simulink library "halin"  (R2021b)
settings: Solver=VariableStepAuto  StartTime=0.0  StopTime=10.0  RelTol=1e-3
undefined symbols (not defined in the file): KHAL_CAN1ABM1E2E_flg, KHAL_CAN1ESC1E2E_flg, KHAL_CAN1ESC5E2E_flg, KHAL_CAN1ESC7E2E_flg, KHAL_CAN1FCM2E2E_flg, KHAL_CAN1FCM3E2E_flg, KHAL_CAN1FCM4E2E_flg, KHAL_CAN3BMS1E2E_flg, KHAL_CAN3BMS6E2E_flg, KHAL_CAN3CCU1E2E_flg, KHAL_CAN3CCU2E2E_flg, KHAL_CAN3MCUF1E2E_flg, KHAL_CAN3MCUR1E2E_flg, KHAL_CAN3Shifter1E2E_flg, TRUE
libraries: simulink x420, FVT_lib x149, hcu_lib x49
(part 11 of 14)

== system halin/HAL_IN/CAN4/GW_ZoneDR1 ==
  DT_CAN4_SG_GW_ZoneDR1 : Inport
  CSWDimSw : Subsystem
  CSWFWasSwSta : Subsystem
  CSWFWipSwSta : Subsystem
  CSWPassSWSta : Subsystem
  CSWRWasSWSta : Subsystem
  CSWRWipIntSwSta : Subsystem
  CSWTurnSwSta : Subsystem
  DrLockSta : Subsystem
  MIRRORFOLDSW : Subsystem
  RLSLampSta : Subsystem
  RLSRainSnrWiperCmd : Subsystem
  RLTurnLampC : Subsystem
  RRTurnLampC : Subsystem
  RWiperAS : Subsystem
  RWiperProtection : Subsystem
  bus_selector : BusSelector  OutputSignals=CAN4_CSW_DimSw
  bus_selector1 : BusSelector  OutputSignals=CAN4_CSW_FWasSw_Sta
  bus_selector10 : BusSelector  OutputSignals=CAN4_RLS_RainSnrWiperCmd
  bus_selector11 : BusSelector  OutputSignals=CAN4_RLTurnLampC
  bus_selector12 : BusSelector  OutputSignals=CAN4_RRTurnLampC
  bus_selector13 : BusSelector  OutputSignals=CAN4_RWiperAS
  bus_selector14 : BusSelector  OutputSignals=CAN4_RWiperProtection
  bus_selector2 : BusSelector  OutputSignals=CAN4_CSW_FWipSw_Sta
  bus_selector3 : BusSelector  OutputSignals=CAN4_CSW_PassSW_Sta
  bus_selector4 : BusSelector  OutputSignals=CAN4_CSW_RWasSW_Sta
  bus_selector5 : BusSelector  OutputSignals=CAN4_CSW_RWipIntSw_Sta
  bus_selector6 : BusSelector  OutputSignals=CAN4_CSW_TurnSw_Sta
  bus_selector7 : BusSelector  OutputSignals=CAN4_DrLockSta
  bus_selector8 : BusSelector  OutputSignals=CAN4_MIRROR_FOLD_SW
  bus_selector9 : BusSelector  OutputSignals=CAN4_RLS_Lamp_Sta
  VHAL_CSWDimSw_flg : Outport
  VHAL_CSWFWasSwSta_enum : Outport  Port=2
  VHAL_CSWFWipSwSta_enum : Outport  Port=3
  VHAL_CSWPassSWSta_flg : Outport  Port=4
  VHAL_CSWRWasSWSta_enum : Outport  Port=5
  VHAL_CSWRWipIntSwSta_enum : Outport  Port=6
  VHAL_CSWTurnSwSta_enum : Outport  Port=7
  VHAL_DrLockSta_flg : Outport  Port=8
  VHAL_MIRRORFOLDSW_flg : Outport  Port=9
  VHAL_RLSLampSta_flg : Outport  Port=10
  VHAL_RLSRainSnrWiperCmd_enum : Outport  Port=11
  VHAL_RLTurnLampC_mA : Outport  Port=12
  VHAL_RRTurnLampC_mA : Outport  Port=13
  VHAL_RWiperAS_flg : Outport  Port=14
  VHAL_RWiperProtection_flg : Outport  Port=15
  wires:
  DT_CAN4_SG_GW_ZoneDR1/1 -> [DT_CAN4_SG_GW_ZoneDR1]
  [DT_CAN4_SG_GW_ZoneDR1] -> bus_selector/1
  bus_selector/1 -> CSWDimSw/1(CSW_DimSw)  "<CAN4_CSW_DimSw>"
  CSWDimSw/1(VHAL_CSWDimSw_flg) -> VHAL_CSWDimSw_flg/1
  [DT_CAN4_SG_GW_ZoneDR1] -> bus_selector1/1
  bus_selector1/1 -> CSWFWasSwSta/1(CSW_FWasSw_Sta)  "<CAN4_CSW_FWasSw_Sta>"
  CSWFWasSwSta/1(VHAL_CSWFWasSwSta_enum) -> VHAL_CSWFWasSwSta_enum/1
  [DT_CAN4_SG_GW_ZoneDR1] -> bus_selector2/1
  bus_selector2/1 -> CSWFWipSwSta/1(CSW_FWipSw_Sta)  "<CAN4_CSW_FWipSw_Sta>"
  CSWFWipSwSta/1(VHAL_CSWFWipSwSta_enum) -> VHAL_CSWFWipSwSta_enum/1
  [DT_CAN4_SG_GW_ZoneDR1] -> bus_selector3/1
  bus_selector3/1 -> CSWPassSWSta/1(CSW_PassSW_Sta)  "<CAN4_CSW_PassSW_Sta>"
  CSWPassSWSta/1(VHAL_CSWPassSWSta_flg) -> VHAL_CSWPassSWSta_flg/1
  [DT_CAN4_SG_GW_ZoneDR1] -> bus_selector4/1
  bus_selector4/1 -> CSWRWasSWSta/1(CSW_RWasSW_Sta)  "<CAN4_CSW_RWasSW_Sta>"
  CSWRWasSWSta/1(VHAL_CSWRWasSWSta_enum) -> VHAL_CSWRWasSWSta_enum/1
  [DT_CAN4_SG_GW_ZoneDR1] -> bus_selector5/1
  bus_selector5/1 -> CSWRWipIntSwSta/1(CSW_RWipIntSw_Sta)  "<CAN4_CSW_RWipIntSw_Sta>"
  CSWRWipIntSwSta/1(VHAL_CSWRWipIntSwSta_enum) -> VHAL_CSWRWipIntSwSta_enum/1
  [DT_CAN4_SG_GW_ZoneDR1] -> bus_selector6/1
  bus_selector6/1 -> CSWTurnSwSta/1(CSW_TurnSw_Sta)  "<CAN4_CSW_TurnSw_Sta>"
  CSWTurnSwSta/1(VHAL_CSWTurnSwSta_enum) -> VHAL_CSWTurnSwSta_enum/1
  [DT_CAN4_SG_GW_ZoneDR1] -> bus_selector7/1
  bus_selector7/1 -> DrLockSta/1(DrLockSta)  "<CAN4_DrLockSta>"
  DrLockSta/1(VHAL_DrLockSta_flg) -> VHAL_DrLockSta_flg/1
  [DT_CAN4_SG_GW_ZoneDR1] -> bus_selector8/1
  bus_selector8/1 -> MIRRORFOLDSW/1(MIRROR_FOLD_SW)  "<CAN4_MIRROR_FOLD_SW>"
  MIRRORFOLDSW/1(VHAL_MIRRORFOLDSW_flg) -> VHAL_MIRRORFOLDSW_flg/1
  [DT_CAN4_SG_GW_ZoneDR1] -> bus_selector9/1
  bus_selector9/1 -> RLSLampSta/1(RLS_Lamp_Sta)  "<CAN4_RLS_Lamp_Sta>"
  RLSLampSta/1(VHAL_RLSLampSta_flg) -> VHAL_RLSLampSta_flg/1
  [DT_CAN4_SG_GW_ZoneDR1] -> bus_selector10/1
  bus_selector10/1 -> RLSRainSnrWiperCmd/1(RLS_RainSnrWiperCmd)  "<CAN4_RLS_RainSnrWiperCmd>"
  RLSRainSnrWiperCmd/1(VHAL_RLSRainSnrWiperCmd_enum) -> VHAL_RLSRainSnrWiperCmd_enum/1
  [DT_CAN4_SG_GW_ZoneDR1] -> bus_selector11/1
  bus_selector11/1 -> RLTurnLampC/1(RLTurnLampC)  "<CAN4_RLTurnLampC>"
  RLTurnLampC/1(VHAL_RLTurnLampC_mA) -> VHAL_RLTurnLampC_mA/1
  [DT_CAN4_SG_GW_ZoneDR1] -> bus_selector12/1
  bus_selector12/1 -> RRTurnLampC/1(RRTurnLampC)  "<CAN4_RRTurnLampC>"
  RRTurnLampC/1(VHAL_RRTurnLampC_mA) -> VHAL_RRTurnLampC_mA/1
  [DT_CAN4_SG_GW_ZoneDR1] -> bus_selector13/1
  bus_selector13/1 -> RWiperAS/1(RWiperAS)  "<CAN4_RWiperAS>"
  RWiperAS/1(VHAL_RWiperAS_flg) -> VHAL_RWiperAS_flg/1
  [DT_CAN4_SG_GW_ZoneDR1] -> bus_selector14/1
  bus_selector14/1 -> RWiperProtection/1(RWiperProtection)  "<CAN4_RWiperProtection>"
  RWiperProtection/1(VHAL_RWiperProtection_flg) -> VHAL_RWiperProtection_flg/1

== system halin/HAL_IN/CAN4/GW_ZoneDR2 ==
  DT_CAN4_SG_GW_ZoneDR2 : Inport
  SWCCANCELSta : Subsystem
  SWCResUpSta : Subsystem
  SWCSetdownSta : Subsystem
  SWCmodeSta : Subsystem
  bus_selector : BusSelector  OutputSignals=CAN4_SWC_CANCEL_Sta
  bus_selector1 : BusSelector  OutputSignals=CAN4_SWC_Res_Up_Sta
  bus_selector2 : BusSelector  OutputSignals=CAN4_SWC_Set_down_Sta
  bus_selector3 : BusSelector  OutputSignals=CAN4_SWC_mode_Sta
  VHAL_SWCCANCELSta_flg : Outport
  VHAL_SWCResUpSta_flg : Outport  Port=2
  VHAL_SWCSetdownSta_flg : Outport  Port=3
  VHAL_SWCmodeSta_flg : Outport  Port=4
  wires:
  DT_CAN4_SG_GW_ZoneDR2/1 -> [DT_CAN4_SG_GW_ZoneDR2]
  [DT_CAN4_SG_GW_ZoneDR2] -> bus_selector/1
  bus_selector/1 -> SWCCANCELSta/1(SWC_CANCEL_Sta)  "<CAN4_SWC_CANCEL_Sta>"
  SWCCANCELSta/1(VHAL_SWCCANCELSta_flg) -> VHAL_SWCCANCELSta_flg/1
  [DT_CAN4_SG_GW_ZoneDR2] -> bus_selector1/1
  bus_selector1/1 -> SWCResUpSta/1(SWC_Res_Up_Sta)  "<CAN4_SWC_Res_Up_Sta>"
  SWCResUpSta/1(VHAL_SWCResUpSta_flg) -> VHAL_SWCResUpSta_flg/1
  [DT_CAN4_SG_GW_ZoneDR2] -> bus_selector2/1
  bus_selector2/1 -> SWCSetdownSta/1(SWC_Set_down_Sta)  "<CAN4_SWC_Set_down_Sta>"
  SWCSetdownSta/1(VHAL_SWCSetdownSta_flg) -> VHAL_SWCSetdownSta_flg/1
  [DT_CAN4_SG_GW_ZoneDR2] -> bus_selector3/1
  bus_selector3/1 -> SWCmodeSta/1(SWC_mode_Sta)  "<CAN4_SWC_mode_Sta>"
  SWCmodeSta/1(VHAL_SWCmodeSta_flg) -> VHAL_SWCmodeSta_flg/1

== system halin/HAL_IN/CAN4/GW_ZoneDR3 ==
  DT_CAN4_SG_GW_ZoneDR3 : Inport
  LDrvValWdwOpened : Subsystem
  LPasValWdwOpened : Subsystem
  bus_selector : BusSelector  OutputSignals=CAN4_L_Drv_Val_Wdw_Opened
  bus_selector1 : BusSelector  OutputSignals=CAN4_L_Pas_Val_Wdw_Opened
  VHAL_LDrvValWdwOpened_pct : Outport
  VHAL_LPasValWdwOpened_pct : Outport  Port=2
  wires:
  DT_CAN4_SG_GW_ZoneDR3/1 -> [DT_CAN4_SG_GW_ZoneDR3]
  [DT_CAN4_SG_GW_ZoneDR3] -> bus_selector/1
  bus_selector/1 -> LDrvValWdwOpened/1(L_Drv_Val_Wdw_Opened)  "<CAN4_L_Drv_Val_Wdw_Opened>"
  LDrvValWdwOpened/1(VHAL_LDrvValWdwOpened_pct) -> VHAL_LDrvValWdwOpened_pct/1
  [DT_CAN4_SG_GW_ZoneDR3] -> bus_selector1/1
  bus_selector1/1 -> LPasValWdwOpened/1(L_Pas_Val_Wdw_Opened)  "<CAN4_L_Pas_Val_Wdw_Opened>"
  LPasValWdwOpened/1(VHAL_LPasValWdwOpened_pct) -> VHAL_LPasValWdwOpened_pct/1

== system halin/HAL_IN/CAN4/GW_ZoneDR4 ==
  DT_CAN4_SG_GW_ZoneDR4 : Inport
  LRLDValWdwOpened : Subsystem
  LRRDValWdwOpened : Subsystem
  PTGInnerSW2 : Subsystem
  bus_selector : BusSelector  OutputSignals=CAN4_L_RLD_Val_Wdw_Opened
  bus_selector1 : BusSelector  OutputSignals=CAN4_L_RRD_Val_Wdw_Opened
  bus_selector2 : BusSelector  OutputSignals=CAN4_PTG_Inner_SW_2
  VHAL_LRLDValWdwOpened_pct : Outport
  VHAL_LRRDValWdwOpened_pct : Outport  Port=2
  VHAL_PTGInnerSW2_enum : Outport  Port=3
  wires:
  DT_CAN4_SG_GW_ZoneDR4/1 -> [DT_CAN4_SG_GW_ZoneDR4]
  [DT_CAN4_SG_GW_ZoneDR4] -> bus_selector/1
  bus_selector/1 -> LRLDValWdwOpened/1(L_RLD_Val_Wdw_Opened)  "<CAN4_L_RLD_Val_Wdw_Opened>"
  LRLDValWdwOpened/1(VHAL_LRLDValWdwOpened_pct) -> VHAL_LRLDValWdwOpened_pct/1
  [DT_CAN4_SG_GW_ZoneDR4] -> bus_selector1/1
  bus_selector1/1 -> LRRDValWdwOpened/1(L_RRD_Val_Wdw_Opened)  "<CAN4_L_RRD_Val_Wdw_Opened>"
  LRRDValWdwOpened/1(VHAL_LRRDValWdwOpened_pct) -> VHAL_LRRDValWdwOpened_pct/1
  [DT_CAN4_SG_GW_ZoneDR4] -> bus_selector2/1
  bus_selector2/1 -> PTGInnerSW2/1(PTG_Inner_SW_2)  "<CAN4_PTG_Inner_SW_2>"
  PTGInnerSW2/1(VHAL_PTGInnerSW2_enum) -> VHAL_PTGInnerSW2_enum/1

== system halin/HAL_IN/CAN4/GW_ZoneDR6 ==
  DT_CAN4_SG_GW_ZoneDR6 : Inport
  FrntPTCRearLeActHeatPwr : Subsystem
  FrntPTCRearRiActHeatPwr : Subsystem
  FrntPTCRiActHeatPwr : Subsystem
  bus_selector : BusSelector  OutputSignals=CAN4_FrntPTCRearLeActHeatPwr
  bus_selector1 : BusSelector  OutputSignals=CAN4_FrntPTCRearRiActHeatPwr
  bus_selector2 : BusSelector  OutputSignals=CAN4_FrntPTCRiActHeatPwr
  VHAL_FrntPTCRearLeActHeatPwr_W : Outport
  VHAL_FrntPTCRearRiActHeatPwr_W : Outport  Port=2
  VHAL_FrntPTCRiActHeatPwr_W : Outport  Port=3
  wires:
  DT_CAN4_SG_GW_ZoneDR6/1 -> [DT_CAN4_SG_GW_ZoneDR6]
  [DT_CAN4_SG_GW_ZoneDR6] -> bus_selector/1
  bus_selector/1 -> FrntPTCRearLeActHeatPwr/1(FrntPTCRearLeActHeatPwr)  "<CAN4_FrntPTCRearLeActHeatPwr>"
  FrntPTCRearLeActHeatPwr/1(VHAL_FrntPTCRearLeActHeatPwr_W) -> VHAL_FrntPTCRearLeActHeatPwr_W/1
  [DT_CAN4_SG_GW_ZoneDR6] -> bus_selector1/1
  bus_selector1/1 -> FrntPTCRearRiActHeatPwr/1(FrntPTCRearRiActHeatPwr)  "<CAN4_FrntPTCRearRiActHeatPwr>"
  FrntPTCRearRiActHeatPwr/1(VHAL_FrntPTCRearRiActHeatPwr_W) -> VHAL_FrntPTCRearRiActHeatPwr_W/1
  [DT_CAN4_SG_GW_ZoneDR6] -> bus_selector2/1
  bus_selector2/1 -> FrntPTCRiActHeatPwr/1(FrntPTCRiActHeatPwr)  "<CAN4_FrntPTCRiActHeatPwr>"
  FrntPTCRiActHeatPwr/1(VHAL_FrntPTCRiActHeatPwr_W) -> VHAL_FrntPTCRiActHeatPwr_W/1

== system halin/HAL_IN/CAN4/GW_ZoneFR1 ==
  DT_CAN4_SG_GW_ZoneFR1 : Inport
  FLTurnLampC : Subsystem
  FRTurnLampC : Subsystem
  FWiperAS : Subsystem
  FWiperProtection : Subsystem
  bus_selector : BusSelector  OutputSignals=CAN4_FLTurnLampC
  bus_selector1 : BusSelector  OutputSignals=CAN4_FRTurnLampC
  bus_selector2 : BusSelector  OutputSignals=CAN4_FWiperAS
  bus_selector3 : BusSelector  OutputSignals=CAN4_FWiperProtection
  VHAL_FLTurnLampC_mA : Outport
  VHAL_FRTurnLampC_mA : Outport  Port=2
  VHAL_FWiperAS_flg : Outport  Port=3
  VHAL_FWiperProtection_flg : Outport  Port=4
  wires:
  DT_CAN4_SG_GW_ZoneFR1/1 -> [DT_CAN4_SG_GW_ZoneFR1]
  [DT_CAN4_SG_GW_ZoneFR1] -> bus_selector/1
  bus_selector/1 -> FLTurnLampC/1(FLTurnLampC)  "<CAN4_FLTurnLampC>"
  FLTurnLampC/1(VHAL_FLTurnLampC_mA) -> VHAL_FLTurnLampC_mA/1
  [DT_CAN4_SG_GW_ZoneFR1] -> bus_selector1/1
  bus_selector1/1 -> FRTurnLampC/1(FRTurnLampC)  "<CAN4_FRTurnLampC>"
  FRTurnLampC/1(VHAL_FRTurnLampC_mA) -> VHAL_FRTurnLampC_mA/1
  [DT_CAN4_SG_GW_ZoneFR1] -> bus_selector2/1
  bus_selector2/1 -> FWiperAS/1(FWiperAS)  "<CAN4_FWiperAS>"
  FWiperAS/1(VHAL_FWiperAS_flg) -> VHAL_FWiperAS_flg/1
  [DT_CAN4_SG_GW_ZoneFR1] -> bus_selector3/1
  bus_selector3/1 -> FWiperProtection/1(FWiperProtection)  "<CAN4_FWiperProtection>"
  FWiperProtection/1(VHAL_FWiperProtection_flg) -> VHAL_FWiperProtection_flg/1

== system halin/HAL_IN/CAN4/GW_ZoneFR2 ==
  DT_CAN4_SG_GW_ZoneFR2 : Inport
  COMPStatorSpd : Subsystem
  CompProEN : Subsystem
  bus_selector : BusSelector  OutputSignals=CAN4_COMP_StatorSpd
  bus_selector1 : BusSelector  OutputSignals=CAN4_CompProEN
  VHAL_COMPStatorSpd_rpm : Outport
  VHAL_CompProEN_flg : Outport  Port=2
  wires:
  DT_CAN4_SG_GW_ZoneFR2/1 -> [DT_CAN4_SG_GW_ZoneFR2]
  [DT_CAN4_SG_GW_ZoneFR2] -> bus_selector/1
  bus_selector/1 -> COMPStatorSpd/1(COMP_StatorSpd)  "<CAN4_COMP_StatorSpd>"
  COMPStatorSpd/1(VHAL_COMPStatorSpd_rpm) -> VHAL_COMPStatorSpd_rpm/1
  [DT_CAN4_SG_GW_ZoneFR2] -> bus_selector1/1
  bus_selector1/1 -> CompProEN/1(CompProEN)  "<CAN4_CompProEN>"
  CompProEN/1(VHAL_CompProEN_flg) -> VHAL_CompProEN_flg/1

== system halin/HAL_IN/CAN4/VHAL_CANMsgInvalidDKC1_flg ==
  Cast To Boolean13 : DataTypeConversion  OutDataTypeStr=boolean
  Constant : Constant  Value=TRUE
  Latch13 : hcu_lib/Basic_Blocks/Latch
  Switch13 : Switch  Criteria=u2 ~= 0
  Unit Delay : UnitDelay  SampleTime=-1  HasFrameUpgradeWarning=on
  UnitConverter : DataTypeConversion  OutDataTypeStr=boolean
  Out : Outport
  wires:
  Constant/1 -> Switch13/3
  Unit Delay/1 -> Cast To Boolean13/1
  Cast To Boolean13/1 -> Switch13/1, Latch13/1
  Switch13/1 -> UnitConverter/1
  Latch13/1 -> Switch13/2
  UnitConverter/1 -> Unit Delay/1, Out/1  "VHAL_CANMsgInvalidDKC1_flg"

== system halin/HAL_IN/CAN4/VHAL_CANMsgInvalidDKC2_flg ==
  Cast To Boolean13 : DataTypeConversion  OutDataTypeStr=boolean
  Constant : Constant  Value=TRUE
  Latch13 : hcu_lib/Basic_Blocks/Latch
  Switch13 : Switch  Criteria=u2 ~= 0
  Unit Delay : UnitDelay  SampleTime=-1  HasFrameUpgradeWarning=on
  UnitConverter : DataTypeConversion  OutDataTypeStr=boolean
  Out : Outport
  wires:
  Constant/1 -> Switch13/3
  Unit Delay/1 -> Cast To Boolean13/1
  Cast To Boolean13/1 -> Switch13/1, Latch13/1
  Switch13/1 -> UnitConverter/1
  Latch13/1 -> Switch13/2
  UnitConverter/1 -> Unit Delay/1, Out/1  "VHAL_CANMsgInvalidDKC2_flg"

== system halin/HAL_IN/CAN4/VHAL_CANMsgInvalidGWZDRPTG1_flg ==
  Cast To Boolean13 : DataTypeConversion  OutDataTypeStr=boolean
  Constant : Constant  Value=TRUE
  Latch13 : hcu_lib/Basic_Blocks/Latch
  Switch13 : Switch  Criteria=u2 ~= 0
  Unit Delay : UnitDelay  SampleTime=-1  HasFrameUpgradeWarning=on
  UnitConverter : DataTypeConversion  OutDataTypeStr=boolean
  Out : Outport
  wires:
  Constant/1 -> Switch13/3
  Unit Delay/1 -> Cast To Boolean13/1
  Cast To Boolean13/1 -> Switch13/1, Latch13/1
  Switch13/1 -> UnitConverter/1
  Latch13/1 -> Switch13/2
  UnitConverter/1 -> Unit Delay/1, Out/1  "VHAL_CANMsgInvalidGWZDRPTG1_flg"

== system halin/HAL_IN/CAN4/VHAL_CANMsgInvalidGWZoneDR1_flg ==
  Cast To Boolean13 : DataTypeConversion  OutDataTypeStr=boolean
  Constant : Constant  Value=TRUE
  Latch13 : hcu_lib/Basic_Blocks/Latch
  Switch13 : Switch  Criteria=u2 ~= 0
  Unit Delay : UnitDelay  SampleTime=-1  HasFrameUpgradeWarning=on
  UnitConverter : DataTypeConversion  OutDataTypeStr=boolean
  Out : Outport
  wires:
  Constant/1 -> Switch13/3
  Unit Delay/1 -> Cast To Boolean13/1
  Cast To Boolean13/1 -> Switch13/1, Latch13/1
  Switch13/1 -> UnitConverter/1
  Latch13/1 -> Switch13/2
  UnitConverter/1 -> Unit Delay/1, Out/1  "VHAL_CANMsgInvalidGWZoneDR1_flg"

== system halin/HAL_IN/CAN4/VHAL_CANMsgInvalidGWZoneDR2_flg ==
  Cast To Boolean13 : DataTypeConversion  OutDataTypeStr=boolean
  Constant : Constant  Value=TRUE
  Latch13 : hcu_lib/Basic_Blocks/Latch
  Switch13 : Switch  Criteria=u2 ~= 0
  Unit Delay : UnitDelay  SampleTime=-1  HasFrameUpgradeWarning=on
  UnitConverter : DataTypeConversion  OutDataTypeStr=boolean
  Out : Outport
  wires:
  Constant/1 -> Switch13/3
  Unit Delay/1 -> Cast To Boolean13/1
  Cast To Boolean13/1 -> Switch13/1, Latch13/1
  Switch13/1 -> UnitConverter/1
  Latch13/1 -> Switch13/2
  UnitConverter/1 -> Unit Delay/1, Out/1  "VHAL_CANMsgInvalidGWZoneDR2_flg"

== system halin/HAL_IN/CAN4/VHAL_CANMsgInvalidGWZoneDR3_flg ==
  Cast To Boolean13 : DataTypeConversion  OutDataTypeStr=boolean
  Constant : Constant  Value=TRUE
  Latch13 : hcu_lib/Basic_Blocks/Latch
  Switch13 : Switch  Criteria=u2 ~= 0
  Unit Delay : UnitDelay  SampleTime=-1  HasFrameUpgradeWarning=on
  UnitConverter : DataTypeConversion  OutDataTypeStr=boolean
  Out : Outport
  wires:
  Constant/1 -> Switch13/3
  Unit Delay/1 -> Cast To Boolean13/1
  Cast To Boolean13/1 -> Switch13/1, Latch13/1
  Switch13/1 -> UnitConverter/1
  Latch13/1 -> Switch13/2
  UnitConverter/1 -> Unit Delay/1, Out/1  "VHAL_CANMsgInvalidGWZoneDR3_flg"

== system halin/HAL_IN/CAN4/VHAL_CANMsgInvalidGWZoneDR4_flg ==
  Cast To Boolean13 : DataTypeConversion  OutDataTypeStr=boolean
  Constant : Constant  Value=TRUE
  Latch13 : hcu_lib/Basic_Blocks/Latch
  Switch13 : Switch  Criteria=u2 ~= 0
  Unit Delay : UnitDelay  SampleTime=-1  HasFrameUpgradeWarning=on
  UnitConverter : DataTypeConversion  OutDataTypeStr=boolean
  Out : Outport
  wires:
  Constant/1 -> Switch13/3
  Unit Delay/1 -> Cast To Boolean13/1
  Cast To Boolean13/1 -> Switch13/1, Latch13/1
  Switch13/1 -> UnitConverter/1
  Latch13/1 -> Switch13/2
  UnitConverter/1 -> Unit Delay/1, Out/1  "VHAL_CANMsgInvalidGWZoneDR4_flg"

== system halin/HAL_IN/CAN4/VHAL_CANMsgInvalidGWZoneDR6_flg ==
  Cast To Boolean13 : DataTypeConversion  OutDataTypeStr=boolean
  Constant : Constant  Value=TRUE
  Latch13 : hcu_lib/Basic_Blocks/Latch
  Switch13 : Switch  Criteria=u2 ~= 0
  Unit Delay : UnitDelay  SampleTime=-1  HasFrameUpgradeWarning=on
  UnitConverter : DataTypeConversion  OutDataTypeStr=boolean
  Out : Outport
  wires:
  Constant/1 -> Switch13/3
  Unit Delay/1 -> Cast To Boolean13/1
  Cast To Boolean13/1 -> Switch13/1, Latch13/1
  Switch13/1 -> UnitConverter/1
  Latch13/1 -> Switch13/2
  UnitConverter/1 -> Unit Delay/1, Out/1  "VHAL_CANMsgInvalidGWZoneDR6_flg"

== system halin/HAL_IN/CAN4/VHAL_CANMsgInvalidGWZoneFR1_flg ==
  Cast To Boolean13 : DataTypeConversion  OutDataTypeStr=boolean
  Constant : Constant  Value=TRUE
  Latch13 : hcu_lib/Basic_Blocks/Latch
  Switch13 : Switch  Criteria=u2 ~= 0
  Unit Delay : UnitDelay  SampleTime=-1  HasFrameUpgradeWarning=on
  UnitConverter : DataTypeConversion  OutDataTypeStr=boolean
  Out : Outport
  wires:
  Constant/1 -> Switch13/3
  Unit Delay/1 -> Cast To Boolean13/1
  Cast To Boolean13/1 -> Switch13/1, Latch13/1
  Switch13/1 -> UnitConverter/1
  Latch13/1 -> Switch13/2
  UnitConverter/1 -> Unit Delay/1, Out/1  "VHAL_CANMsgInvalidGWZoneFR1_flg"

== system halin/HAL_IN/CAN4/VHAL_CANMsgInvalidGWZoneFR2_flg ==
  Cast To Boolean13 : DataTypeConversion  OutDataTypeStr=boolean
  Constant : Constant  Value=TRUE
  Latch13 : hcu_lib/Basic_Blocks/Latch
  Switch13 : Switch  Criteria=u2 ~= 0
  Unit Delay : UnitDelay  SampleTime=-1  HasFrameUpgradeWarning=on
  UnitConverter : DataTypeConversion  OutDataTypeStr=boolean
  Out : Outport
  wires:
  Constant/1 -> Switch13/3
  Unit Delay/1 -> Cast To Boolean13/1
  Cast To Boolean13/1 -> Switch13/1, Latch13/1
  Switch13/1 -> UnitConverter/1
  Latch13/1 -> Switch13/2
  UnitConverter/1 -> Unit Delay/1, Out/1  "VHAL_CANMsgInvalidGWZoneFR2_flg"

== system halin/HAL_IN/CAN4/VHAL_CANMsgInvalidZoneDrSCP_flg ==
  Cast To Boolean13 : DataTypeConversion  OutDataTypeStr=boolean
  Constant : Constant  Value=TRUE
  Latch13 : hcu_lib/Basic_Blocks/Latch
  Switch13 : Switch  Criteria=u2 ~= 0
  Unit Delay : UnitDelay  SampleTime=-1  HasFrameUpgradeWarning=on
  UnitConverter : DataTypeConversion  OutDataTypeStr=boolean
  Out : Outport
  wires:
  Constant/1 -> Switch13/3
  Unit Delay/1 -> Cast To Boolean13/1
  Cast To Boolean13/1 -> Switch13/1, Latch13/1
  Switch13/1 -> UnitConverter/1
  Latch13/1 -> Switch13/2
  UnitConverter/1 -> Unit Delay/1, Out/1  "VHAL_CANMsgInvalidZoneDrSCP_flg"

== system halin/HAL_IN/CAN4/VHAL_CANMsgInvalidZoneDrTHCM_flg ==
  Cast To Boolean13 : DataTypeConversion  OutDataTypeStr=boolean
  Constant : Constant  Value=TRUE
  Latch13 : hcu_lib/Basic_Blocks/Latch
  Switch13 : Switch  Criteria=u2 ~= 0
  Unit Delay : UnitDelay  SampleTime=-1  HasFrameUpgradeWarning=on
  UnitConverter : DataTypeConversion  OutDataTypeStr=boolean
  Out : Outport
  wires:
  Constant/1 -> Switch13/3
  Unit Delay/1 -> Cast To Boolean13/1
  Cast To Boolean13/1 -> Switch13/1, Latch13/1
  Switch13/1 -> UnitConverter/1
  Latch13/1 -> Switch13/2
  UnitConverter/1 -> Unit Delay/1, Out/1  "VHAL_CANMsgInvalidZoneDrTHCM_flg"

== system halin/HAL_IN/CAN4/VHAL_CANMsgInvalidZoneDrVCU_flg ==
  Cast To Boolean13 : DataTypeConversion  OutDataTypeStr=boolean
  Constant : Constant  Value=TRUE
  Latch13 : hcu_lib/Basic_Blocks/Latch
  Switch13 : Switch  Criteria=u2 ~= 0
  Unit Delay : UnitDelay  SampleTime=-1  HasFrameUpgradeWarning=on
  UnitConverter : DataTypeConversion  OutDataTypeStr=boolean
  Out : Outport
  wires:
  Constant/1 -> Switch13/3
  Unit Delay/1 -> Cast To Boolean13/1
  Cast To Boolean13/1 -> Switch13/1, Latch13/1
  Switch13/1 -> UnitConverter/1
  Latch13/1 -> Switch13/2
  UnitConverter/1 -> Unit Delay/1, Out/1  "VHAL_CANMsgInvalidZoneDrVCU_flg"

== system halin/HAL_IN/CAN4/VHAL_CANMsgInvalidZoneFrTHCM_flg ==
  Cast To Boolean13 : DataTypeConversion  OutDataTypeStr=boolean
  Constant : Constant  Value=TRUE
  Latch13 : hcu_lib/Basic_Blocks/Latch
  Switch13 : Switch  Criteria=u2 ~= 0
  Unit Delay : UnitDelay  SampleTime=-1  HasFrameUpgradeWarning=on
  UnitConverter : DataTypeConversion  OutDataTypeStr=boolean
  Out : Outport
  wires:
  Constant/1 -> Switch13/3
  Unit Delay/1 -> Cast To Boolean13/1
  Cast To Boolean13/1 -> Switch13/1, Latch13/1
  Switch13/1 -> UnitConverter/1
  Latch13/1 -> Switch13/2
  UnitConverter/1 -> Unit Delay/1, Out/1  "VHAL_CANMsgInvalidZoneFrTHCM_flg"

== system halin/HAL_IN/CAN4/Zone_Dr_SCP ==
  DT_CAN4_SG_Zone_Dr_SCP : Inport
  DrSCPSysErrLmp : Subsystem
  RegenMode : Subsystem
  SetSpd : Subsystem
  ZoneSpdCtrlMode : Subsystem
  bus_selector : BusSelector  OutputSignals=CAN4_DrSCPSysErrLmp
  bus_selector1 : BusSelector  OutputSignals=CAN4_RegenMode
  bus_selector2 : BusSelector  OutputSignals=CAN4_Set_Spd
  bus_selector3 : BusSelector  OutputSignals=CAN4_Zone_Spd_Ctrl_Mode
  VHAL_DrSCPSysErrLmp_flg : Outport
  VHAL_RegenMode_enum : Outport  Port=2
  VHAL_SetSpd_kph : Outport  Port=3
  VHAL_ZoneSpdCtrlMode_enum : Outport  Port=4
  wires:
  DT_CAN4_SG_Zone_Dr_SCP/1 -> [DT_CAN4_SG_Zone_Dr_SCP]
  [DT_CAN4_SG_Zone_Dr_SCP] -> bus_selector/1
  bus_selector/1 -> DrSCPSysErrLmp/1(DrSCPSysErrLmp)  "<CAN4_DrSCPSysErrLmp>"
  DrSCPSysErrLmp/1(VHAL_DrSCPSysErrLmp_flg) -> VHAL_DrSCPSysErrLmp_flg/1
  [DT_CAN4_SG_Zone_Dr_SCP] -> bus_selector1/1
  bus_selector1/1 -> RegenMode/1(RegenMode)  "<CAN4_RegenMode>"
  RegenMode/1(VHAL_RegenMode_enum) -> VHAL_RegenMode_enum/1
  [DT_CAN4_SG_Zone_Dr_SCP] -> bus_selector2/1
  bus_selector2/1 -> SetSpd/1(Set_Spd)  "<CAN4_Set_Spd>"
  SetSpd/1(VHAL_SetSpd_kph) -> VHAL_SetSpd_kph/1
  [DT_CAN4_SG_Zone_Dr_SCP] -> bus_selector3/1
  bus_selector3/1 -> ZoneSpdCtrlMode/1(Zone_Spd_Ctrl_Mode)  "<CAN4_Zone_Spd_Ctrl_Mode>"
  ZoneSpdCtrlMode/1(VHAL_ZoneSpdCtrlMode_enum) -> VHAL_ZoneSpdCtrlMode_enum/1

== system halin/HAL_IN/CAN4/Zone_Dr_THCM ==
  DT_CAN4_SG_Zone_Dr_THCM : Inport
  BlowerErr : Subsystem
  SolarL : Subsystem
  SolarLErr : Subsystem
  SolarR : Subsystem
  SolarRErr : Subsystem
  TFaceL : Subsystem
  TFaceLErr : Subsystem
  TFaceR : Subsystem
  TFaceRErr : Subsystem
  TFaceRr : Subsystem
  TFaceRrErr : Subsystem
  TFootL : Subsystem
  TFootLErr : Subsystem
  TFootR : Subsystem
  TFootRErr : Subsystem
  TFootRr : Subsystem
  TFootRrErr : Subsystem
  Tevap : Subsystem
  TevapErr : Subsystem
  Tincar : Subsystem
  TincarErr : Subsystem
  bus_selector : BusSelector  OutputSignals=CAN4_Blower_Err
  bus_selector1 : BusSelector  OutputSignals=CAN4_SolarL
  bus_selector10 : BusSelector  OutputSignals=CAN4_T_Face_Rr_Err
  bus_selector11 : BusSelector  OutputSignals=CAN4_T_Foot_L
  bus_selector12 : BusSelector  OutputSignals=CAN4_T_Foot_L_Err
  bus_selector13 : BusSelector  OutputSignals=CAN4_T_Foot_R
  bus_selector14 : BusSelector  OutputSignals=CAN4_T_Foot_R_Err
  bus_selector15 : BusSelector  OutputSignals=CAN4_T_Foot_Rr
  bus_selector16 : BusSelector  OutputSignals=CAN4_T_Foot_Rr_Err
  bus_selector17 : BusSelector  OutputSignals=CAN4_Tevap
  bus_selector18 : BusSelector  OutputSignals=CAN4_Tevap_Err
  bus_selector19 : BusSelector  OutputSignals=CAN4_Tincar
  bus_selector2 : BusSelector  OutputSignals=CAN4_SolarL_Err
  bus_selector20 : BusSelector  OutputSignals=CAN4_Tincar_Err
  bus_selector3 : BusSelector  OutputSignals=CAN4_SolarR
  bus_selector4 : BusSelector  OutputSignals=CAN4_SolarR_Err
  bus_selector5 : BusSelector  OutputSignals=CAN4_T_Face_L
  bus_selector6 : BusSelector  OutputSignals=CAN4_T_Face_L_Err
  bus_selector7 : BusSelector  OutputSignals=CAN4_T_Face_R
  bus_selector8 : BusSelector  OutputSignals=CAN4_T_Face_R_Err
  bus_selector9 : BusSelector  OutputSignals=CAN4_T_Face_Rr
  VHAL_BlowerErr_enum : Outport
  VHAL_SolarL_W : Outport  Port=2
  VHAL_SolarLErr_enum : Outport  Port=3
  VHAL_SolarR_W : Outport  Port=4
  VHAL_SolarRErr_enum : Outport  Port=5
  VHAL_TFaceL_C : Outport  Port=6
  VHAL_TFaceLErr_enum : Outport  Port=7
  VHAL_TFaceR_C : Outport  Port=8
  VHAL_TFaceRErr_enum : Outport  Port=9
  VHAL_TFaceRr_C : Outport  Port=10
  VHAL_TFaceRrErr_enum : Outport  Port=11
  VHAL_TFootL_C : Outport  Port=12
  VHAL_TFootLErr_enum : Outport  Port=13
  VHAL_TFootR_C : Outport  Port=14
  VHAL_TFootRErr_enum : Outport  Port=15
  VHAL_TFootRr_C : Outport  Port=16
  VHAL_TFootRrErr_enum : Outport  Port=17
  VHAL_Tevap_C : Outport  Port=18
  VHAL_TevapErr_enum : Outport  Port=19
  VHAL_Tincar_C : Outport  Port=20
  VHAL_TincarErr_enum : Outport  Port=21
  wires:
  DT_CAN4_SG_Zone_Dr_THCM/1 -> [DT_CAN4_SG_Zone_Dr_THCM]
  [DT_CAN4_SG_Zone_Dr_THCM] -> bus_selector/1
  bus_selector/1 -> BlowerErr/1(Blower_Err)  "<CAN4_Blower_Err>"
  BlowerErr/1(VHAL_BlowerErr_enum) -> VHAL_BlowerErr_enum/1
  [DT_CAN4_SG_Zone_Dr_THCM] -> bus_selector1/1
  bus_selector1/1 -> SolarL/1(SolarL)  "<CAN4_SolarL>"
  SolarL/1(VHAL_SolarL_W) -> VHAL_SolarL_W/1
  [DT_CAN4_SG_Zone_Dr_THCM] -> bus_selector2/1
  bus_selector2/1 -> SolarLErr/1(SolarL_Err)  "<CAN4_SolarL_Err>"
  SolarLErr/1(VHAL_SolarLErr_enum) -> VHAL_SolarLErr_enum/1
  [DT_CAN4_SG_Zone_Dr_THCM] -> bus_selector3/1
  bus_selector3/1 -> SolarR/1(SolarR)  "<CAN4_SolarR>"
  SolarR/1(VHAL_SolarR_W) -> VHAL_SolarR_W/1
  [DT_CAN4_SG_Zone_Dr_THCM] -> bus_selector4/1
  bus_selector4/1 -> SolarRErr/1(SolarR_Err)  "<CAN4_SolarR_Err>"
  SolarRErr/1(VHAL_SolarRErr_enum) -> VHAL_SolarRErr_enum/1
  [DT_CAN4_SG_Zone_Dr_THCM] -> bus_selector5/1
  bus_selector5/1 -> TFaceL/1(T_Face_L)  "<CAN4_T_Face_L>"
  TFaceL/1(VHAL_TFaceL_C) -> VHAL_TFaceL_C/1
  [DT_CAN4_SG_Zone_Dr_THCM] -> bus_selector6/1
  bus_selector6/1 -> TFaceLErr/1(T_Face_L_Err)  "<CAN4_T_Face_L_Err>"
  TFaceLErr/1(VHAL_TFaceLErr_enum) -> VHAL_TFaceLErr_enum/1
  [DT_CAN4_SG_Zone_Dr_THCM] -> bus_selector7/1
  bus_selector7/1 -> TFaceR/1(T_Face_R)  "<CAN4_T_Face_R>"
  TFaceR/1(VHAL_TFaceR_C) -> VHAL_TFaceR_C/1
  [DT_CAN4_SG_Zone_Dr_THCM] -> bus_selector8/1
  bus_selector8/1 -> TFaceRErr/1(T_Face_R_Err)  "<CAN4_T_Face_R_Err>"
  TFaceRErr/1(VHAL_TFaceRErr_enum) -> VHAL_TFaceRErr_enum/1
  [DT_CAN4_SG_Zone_Dr_THCM] -> bus_selector9/1
  bus_selector9/1 -> TFaceRr/1(T_Face_Rr)  "<CAN4_T_Face_Rr>"
  TFaceRr/1(VHAL_TFaceRr_C) -> VHAL_TFaceRr_C/1
  [DT_CAN4_SG_Zone_Dr_THCM] -> bus_selector10/1
  bus_selector10/1 -> TFaceRrErr/1(T_Face_Rr_Err)  "<CAN4_T_Face_Rr_Err>"
  TFaceRrErr/1(VHAL_TFaceRrErr_enum) -> VHAL_TFaceRrErr_enum/1
  [DT_CAN4_SG_Zone_Dr_THCM] -> bus_selector11/1
  bus_selector11/1 -> TFootL/1(T_Foot_L)  "<CAN4_T_Foot_L>"
  TFootL/1(VHAL_TFootL_C) -> VHAL_TFootL_C/1
  [DT_CAN4_SG_Zone_Dr_THCM] -> bus_selector12/1
  bus_selector12/1 -> TFootLErr/1(T_Foot_L_Err)  "<CAN4_T_Foot_L_Err>"
  TFootLErr/1(VHAL_TFootLErr_enum) -> VHAL_TFootLErr_enum/1
  [DT_CAN4_SG_Zone_Dr_THCM] -> bus_selector13/1
  bus_selector13/1 -> TFootR/1(T_Foot_R)  "<CAN4_T_Foot_R>"
  TFootR/1(VHAL_TFootR_C) -> VHAL_TFootR_C/1
  [DT_CAN4_SG_Zone_Dr_THCM] -> bus_selector14/1
  bus_selector14/1 -> TFootRErr/1(T_Foot_R_Err)  "<CAN4_T_Foot_R_Err>"
  TFootRErr/1(VHAL_TFootRErr_enum) -> VHAL_TFootRErr_enum/1
  [DT_CAN4_SG_Zone_Dr_THCM] -> bus_selector15/1
  bus_selector15/1 -> TFootRr/1(T_Foot_Rr)  "<CAN4_T_Foot_Rr>"
  TFootRr/1(VHAL_TFootRr_C) -> VHAL_TFootRr_C/1
  [DT_CAN4_SG_Zone_Dr_THCM] -> bus_selector16/1
  bus_selector16/1 -> TFootRrErr/1(T_Foot_Rr_Err)  "<CAN4_T_Foot_Rr_Err>"
  TFootRrErr/1(VHAL_TFootRrErr_enum) -> VHAL_TFootRrErr_enum/1
  [DT_CAN4_SG_Zone_Dr_THCM] -> bus_selector17/1
  bus_selector17/1 -> Tevap/1(Tevap)  "<CAN4_Tevap>"
  Tevap/1(VHAL_Tevap_C) -> VHAL_Tevap_C/1
  [DT_CAN4_SG_Zone_Dr_THCM] -> bus_selector18/1
  bus_selector18/1 -> TevapErr/1(Tevap_Err)  "<CAN4_Tevap_Err>"
  TevapErr/1(VHAL_TevapErr_enum) -> VHAL_TevapErr_enum/1
  [DT_CAN4_SG_Zone_Dr_THCM] -> bus_selector19/1
  bus_selector19/1 -> Tincar/1(Tincar)  "<CAN4_Tincar>"
  Tincar/1(VHAL_Tincar_C) -> VHAL_Tincar_C/1
  [DT_CAN4_SG_Zone_Dr_THCM] -> bus_selector20/1
  bus_selector20/1 -> TincarErr/1(Tincar_Err)  "<CAN4_Tincar_Err>"
  TincarErr/1(VHAL_TincarErr_enum) -> VHAL_TincarErr_enum/1

== system halin/HAL_IN/CAN4/Zone_Dr_VCU ==
  DT_CAN4_SG_Zone_Dr_VCU : Inport
  DrAuBoxPwrN1Curr : Subsystem
  DrAuBoxPwrN2Curr : Subsystem
  DrColumnSWFault : Subsystem
  DrCtrlBDVolt : Subsystem
  DrCtrlTemp : Subsystem
  DrEOBDFault : Subsystem
  DrIVIFault : Subsystem
  DrInfoFault : Subsystem
  DrPMMLVOutPErrLmp : Subsystem
  DrPMMLimpHomeActReq : Subsystem
  DrPMMSysErrLmp : Subsystem
  DrPowerTemp1 : Subsystem
  DrPowerTemp2 : Subsystem
  DrPwrInformationSta : Subsystem
  DrPwrONA1Curr : Subsystem
  DrPwrONA2Curr : Subsystem
  DrPwrSta : Subsystem
  DrPwrStdbyACurr : Subsystem
  DrPwrWindowECUFault : Subsystem
  DrStdAErrSta : Subsystem
  DrTHCMFault : Subsystem
  ZoneDrMalfunLevel : Subsystem
  bus_selector : BusSelector  OutputSignals=CAN4_DrAuBoxPwrN1Curr
  bus_selector1 : BusSelector  OutputSignals=CAN4_DrAuBoxPwrN2Curr
  bus_selector10 : BusSelector  OutputSignals=CAN4_DrPMMSysErrLmp
  bus_selector11 : BusSelector  OutputSignals=CAN4_DrPowerTemp1
  bus_selector12 : BusSelector  OutputSignals=CAN4_DrPowerTemp2
  bus_selector13 : BusSelector  OutputSignals=CAN4_DrPwrInformationSta
  bus_selector14 : BusSelector  OutputSignals=CAN4_DrPwrONA1Curr
  bus_selector15 : BusSelector  OutputSignals=CAN4_DrPwrONA2Curr
  bus_selector16 : BusSelector  OutputSignals=CAN4_DrPwrSta
  bus_selector17 : BusSelector  OutputSignals=CAN4_DrPwrStdbyACurr
  bus_selector18 : BusSelector  OutputSignals=CAN4_DrPwrWindowECUFault
  bus_selector19 : BusSelector  OutputSignals=CAN4_DrStdAErrSta
  bus_selector2 : BusSelector  OutputSignals=CAN4_DrColumnSWFault
  bus_selector20 : BusSelector  OutputSignals=CAN4_DrTHCMFault
  bus_selector21 : BusSelector  OutputSignals=CAN4_ZoneDrMalfunLevel
  bus_selector3 : BusSelector  OutputSignals=CAN4_DrCtrlBDVolt
  bus_selector4 : BusSelector  OutputSignals=CAN4_DrCtrlTemp
  bus_selector5 : BusSelector  OutputSignals=CAN4_DrEOBDFault
  bus_selector6 : BusSelector  OutputSignals=CAN4_DrIVIFault
  bus_selector7 : BusSelector  OutputSignals=CAN4_DrInfoFault
  bus_selector8 : BusSelector  OutputSignals=CAN4_DrPMMLVOutPErrLmp
  bus_selector9 : BusSelector  OutputSignals=CAN4_DrPMMLimpHomeActReq
  VHAL_DrAuBoxPwrN1Curr_A : Outport
  VHAL_DrAuBoxPwrN2Curr_A : Outport  Port=2
  VHAL_DrColumnSWFault_enum : Outport  Port=3
  VHAL_DrCtrlBDVolt_V : Outport  Port=4
  VHAL_DrCtrlTemp_C : Outport  Port=5
  VHAL_DrEOBDFault_enum : Outport  Port=6
  VHAL_DrIVIFault_enum : Outport  Port=7
  VHAL_DrInfoFault_enum : Outport  Port=8
  VHAL_DrPMMLVOutPErrLmp_flg : Outport  Port=9
  VHAL_DrPMMLimpHomeActReq_flg : Outport  Port=10
  VHAL_DrPMMSysErrLmp_flg : Outport  Port=11
  VHAL_DrPowerTemp1_C : Outport  Port=12
  VHAL_DrPowerTemp2_C : Outport  Port=13
  VHAL_DrPwrInformationSta_flg : Outport  Port=14
  VHAL_DrPwrONA1Curr_A : Outport  Port=15
  VHAL_DrPwrONA2Curr_A : Outport  Port=16
  VHAL_DrPwrSta_enum : Outport  Port=17
  VHAL_DrPwrStdbyACurr_A : Outport  Port=18
  VHAL_DrPwrWindowECUFault_enum : Outport  Port=19
  VHAL_DrStdAErrSta_flg : Outport  Port=20
  VHAL_DrTHCMFault_enum : Outport  Port=21
  VHAL_ZoneDrMalfunLevel_enum : Outport  Port=22
  wires:
  DT_CAN4_SG_Zone_Dr_VCU/1 -> [DT_CAN4_SG_Zone_Dr_VCU]
  [DT_CAN4_SG_Zone_Dr_VCU] -> bus_selector/1
  bus_selector/1 -> DrAuBoxPwrN1Curr/1(DrAuBoxPwrN1Curr)  "<CAN4_DrAuBoxPwrN1Curr>"
  DrAuBoxPwrN1Curr/1(VHAL_DrAuBoxPwrN1Curr_A) -> VHAL_DrAuBoxPwrN1Curr_A/1
  [DT_CAN4_SG_Zone_Dr_VCU] -> bus_selector1/1
  bus_selector1/1 -> DrAuBoxPwrN2Curr/1(DrAuBoxPwrN2Curr)  "<CAN4_DrAuBoxPwrN2Curr>"
  DrAuBoxPwrN2Curr/1(VHAL_DrAuBoxPwrN2Curr_A) -> VHAL_DrAuBoxPwrN2Curr_A/1
  [DT_CAN4_SG_Zone_Dr_VCU] -> bus_selector2/1
  bus_selector2/1 -> DrColumnSWFault/1(DrColumnSWFault)  "<CAN4_DrColumnSWFault>"
  DrColumnSWFault/1(VHAL_DrColumnSWFault_enum) -> VHAL_DrColumnSWFault_enum/1
  [DT_CAN4_SG_Zone_Dr_VCU] -> bus_selector3/1
  bus_selector3/1 -> DrCtrlBDVolt/1(DrCtrlBDVolt)  "<CAN4_DrCtrlBDVolt>"
  DrCtrlBDVolt/1(VHAL_DrCtrlBDVolt_V) -> VHAL_DrCtrlBDVolt_V/1
  [DT_CAN4_SG_Zone_Dr_VCU] -> bus_selector4/1
  bus_selector4/1 -> DrCtrlTemp/1(DrCtrlTemp)  "<CAN4_DrCtrlTemp>"
  DrCtrlTemp/1(VHAL_DrCtrlTemp_C) -> VHAL_DrCtrlTemp_C/1
  [DT_CAN4_SG_Zone_Dr_VCU] -> bus_selector5/1
  bus_selector5/1 -> DrEOBDFault/1(DrEOBDFault)  "<CAN4_DrEOBDFault>"
  DrEOBDFault/1(VHAL_DrEOBDFault_enum) -> VHAL_DrEOBDFault_enum/1
  [DT_CAN4_SG_Zone_Dr_VCU] -> bus_selector6/1
  bus_selector6/1 -> DrIVIFault/1(DrIVIFault)  "<CAN4_DrIVIFault>"
  DrIVIFault/1(VHAL_DrIVIFault_enum) -> VHAL_DrIVIFault_enum/1
  [DT_CAN4_SG_Zone_Dr_VCU] -> bus_selector7/1
  bus_selector7/1 -> DrInfoFault/1(DrInfoFault)  "<CAN4_DrInfoFault>"
  DrInfoFault/1(VHAL_DrInfoFault_enum) -> VHAL_DrInfoFault_enum/1
  [DT_CAN4_SG_Zone_Dr_VCU] -> bus_selector8/1
  bus_selector8/1 -> DrPMMLVOutPErrLmp/1(DrPMMLVOutPErrLmp)  "<CAN4_DrPMMLVOutPErrLmp>"
  DrPMMLVOutPErrLmp/1(VHAL_DrPMMLVOutPErrLmp_flg) -> VHAL_DrPMMLVOutPErrLmp_flg/1
  [DT_CAN4_SG_Zone_Dr_VCU] -> bus_selector9/1
  bus_selector9/1 -> DrPMMLimpHomeActReq/1(DrPMMLimpHomeActReq)  "<CAN4_DrPMMLimpHomeActReq>"
  DrPMMLimpHomeActReq/1(VHAL_DrPMMLimpHomeActReq_flg) -> VHAL_DrPMMLimpHomeActReq_flg/1
  [DT_CAN4_SG_Zone_Dr_VCU] -> bus_selector10/1
  bus_selector10/1 -> DrPMMSysErrLmp/1(DrPMMSysErrLmp)  "<CAN4_DrPMMSysErrLmp>"
  DrPMMSysErrLmp/1(VHAL_DrPMMSysErrLmp_flg) -> VHAL_DrPMMSysErrLmp_flg/1
  [DT_CAN4_SG_Zone_Dr_VCU] -> bus_selector11/1
  bus_selector11/1 -> DrPowerTemp1/1(DrPowerTemp1)  "<CAN4_DrPowerTemp1>"
  DrPowerTemp1/1(VHAL_DrPowerTemp1_C) -> VHAL_DrPowerTemp1_C/1
  [DT_CAN4_SG_Zone_Dr_VCU] -> bus_selector12/1
  bus_selector12/1 -> DrPowerTemp2/1(DrPowerTemp2)  "<CAN4_DrPowerTemp2>"
  DrPowerTemp2/1(VHAL_DrPowerTemp2_C) -> VHAL_DrPowerTemp2_C/1
  [DT_CAN4_SG_Zone_Dr_VCU] -> bus_selector13/1
  bus_selector13/1 -> DrPwrInformationSta/1(DrPwrInformationSta)  "<CAN4_DrPwrInformationSta>"
  DrPwrInformationSta/1(VHAL_DrPwrInformationSta_flg) -> VHAL_DrPwrInformationSta_flg/1
  [DT_CAN4_SG_Zone_Dr_VCU] -> bus_selector14/1
  bus_selector14/1 -> DrPwrONA1Curr/1(DrPwrONA1Curr)  "<CAN4_DrPwrONA1Curr>"
  DrPwrONA1Curr/1(VHAL_DrPwrONA1Curr_A) -> VHAL_DrPwrONA1Curr_A/1
  [DT_CAN4_SG_Zone_Dr_VCU] -> bus_selector15/1
  bus_selector15/1 -> DrPwrONA2Curr/1(DrPwrONA2Curr)  "<CAN4_DrPwrONA2Curr>"
  DrPwrONA2Curr/1(VHAL_DrPwrONA2Curr_A) -> VHAL_DrPwrONA2Curr_A/1
  [DT_CAN4_SG_Zone_Dr_VCU] -> bus_selector16/1
  bus_selector16/1 -> DrPwrSta/1(DrPwrSta)  "<CAN4_DrPwrSta>"
  DrPwrSta/1(VHAL_DrPwrSta_enum) -> VHAL_DrPwrSta_enum/1
  [DT_CAN4_SG_Zone_Dr_VCU] -> bus_selector17/1
  bus_selector17/1 -> DrPwrStdbyACurr/1(DrPwrStdbyACurr)  "<CAN4_DrPwrStdbyACurr>"
  DrPwrStdbyACurr/1(VHAL_DrPwrStdbyACurr_A) -> VHAL_DrPwrStdbyACurr_A/1
  [DT_CAN4_SG_Zone_Dr_VCU] -> bus_selector18/1
  bus_selector18/1 -> DrPwrWindowECUFault/1(DrPwrWindowECUFault)  "<CAN4_DrPwrWindowECUFault>"
  DrPwrWindowECUFault/1(VHAL_DrPwrWindowECUFault_enum) -> VHAL_DrPwrWindowECUFault_enum/1
  [DT_CAN4_SG_Zone_Dr_VCU] -> bus_selector19/1
  bus_selector19/1 -> DrStdAErrSta/1(DrStdAErrSta)  "<CAN4_DrStdAErrSta>"
  DrStdAErrSta/1(VHAL_DrStdAErrSta_flg) -> VHAL_DrStdAErrSta_flg/1
  [DT_CAN4_SG_Zone_Dr_VCU] -> bus_selector20/1
  bus_selector20/1 -> DrTHCMFault/1(DrTHCMFault)  "<CAN4_DrTHCMFault>"
  DrTHCMFault/1(VHAL_DrTHCMFault_enum) -> VHAL_DrTHCMFault_enum/1
  [DT_CAN4_SG_Zone_Dr_VCU] -> bus_selector21/1
  bus_selector21/1 -> ZoneDrMalfunLevel/1(ZoneDrMalfunLevel)  "<CAN4_ZoneDrMalfunLevel>"
  ZoneDrMalfunLevel/1(VHAL_ZoneDrMalfunLevel_enum) -> VHAL_ZoneDrMalfunLevel_enum/1

== system halin/HAL_IN/CAN4/Zone_Fr_THCM ==
  DT_CAN4_SG_Zone_Fr_THCM : Inport
  AGSErr : Subsystem
  BatInTemp : Subsystem
  BatInTempErr : Subsystem
  BatOutTemp : Subsystem
  COMPErr : Subsystem
  EACProtectEnable : Subsystem
  EWP3Err : Subsystem
  EXV1Err : Subsystem
  EXV2Err : Subsystem
  FanErr : Subsystem
  MotorInTemp : Subsystem
  MotorInTempErr : Subsystem
  MotorOutTemp : Subsystem
  MotorOutTempErr : Subsystem
  PTHighP : Subsystem
  PTHighPErr : Subsystem
  PTHighTact : Subsystem
  PTHighTactErr : Subsystem
  PTLowP1 : Subsystem
  PTLowP1Err : Subsystem
  PTLowP2 : Subsystem
  PTLowP2Err : Subsystem
  PTLowT1 : Subsystem
  PTLowT1Err : Subsystem
  PTLowT2 : Subsystem
  PTLowT2Err : Subsystem
  SOTXVErr : Subsystem
  SOV1Err : Subsystem
  SOV2Err : Subsystem
  SOV3Err : Subsystem
  Tamb : Subsystem
  TambErr : Subsystem
  bus_selector : BusSelector  OutputSignals=CAN4_AGS_Err
  bus_selector1 : BusSelector  OutputSignals=CAN4_Bat_In_Temp
  bus_selector10 : BusSelector  OutputSignals=CAN4_Motor_In_Temp
  bus_selector11 : BusSelector  OutputSignals=CAN4_Motor_In_Temp_Err
  bus_selector12 : BusSelector  OutputSignals=CAN4_Motor_Out_Temp
  bus_selector13 : BusSelector  OutputSignals=CAN4_Motor_Out_Temp_Err
  bus_selector14 : BusSelector  OutputSignals=CAN4_PT_High_P
  bus_selector15 : BusSelector  OutputSignals=CAN4_PT_High_P_Err
  bus_selector16 : BusSelector  OutputSignals=CAN4_PT_High_Tact
  bus_selector17 : BusSelector  OutputSignals=CAN4_PT_High_Tact_Err
  bus_selector18 : BusSelector  OutputSignals=CAN4_PT_Low_P1
  bus_selector19 : BusSelector  OutputSignals=CAN4_PT_Low_P1_Err
  bus_selector2 : BusSelector  OutputSignals=CAN4_Bat_In_Temp_Err
  bus_selector20 : BusSelector  OutputSignals=CAN4_PT_Low_P2
  bus_selector21 : BusSelector  OutputSignals=CAN4_PT_Low_P2_Err
  bus_selector22 : BusSelector  OutputSignals=CAN4_PT_Low_T1
  bus_selector23 : BusSelector  OutputSignals=CAN4_PT_Low_T1_Err
  bus_selector24 : BusSelector  OutputSignals=CAN4_PT_Low_T2
  bus_selector25 : BusSelector  OutputSignals=CAN4_PT_Low_T2_Err
  bus_selector26 : BusSelector  OutputSignals=CAN4_SOTXV_Err
  bus_selector27 : BusSelector  OutputSignals=CAN4_SOV1_Err
  bus_selector28 : BusSelector  OutputSignals=CAN4_SOV2_Err
  bus_selector29 : BusSelector  OutputSignals=CAN4_SOV3_Err
  bus_selector3 : BusSelector  OutputSignals=CAN4_Bat_Out_Temp
  bus_selector30 : BusSelector  OutputSignals=CAN4_Tamb
  bus_selector31 : BusSelector  OutputSignals=CAN4_Tamb_Err
  bus_selector4 : BusSelector  OutputSignals=CAN4_COMP_Err
  bus_selector5 : BusSelector  OutputSignals=CAN4_EACProtectEnable
  bus_selector6 : BusSelector  OutputSignals=CAN4_EWP3_Err
  bus_selector7 : BusSelector  OutputSignals=CAN4_EXV1_Err
  bus_selector8 : BusSelector  OutputSignals=CAN4_EXV2_Err
  bus_selector9 : BusSelector  OutputSignals=CAN4_Fan_Err
  VHAL_AGSErr_enum : Outport
  VHAL_BatInTemp_C : Outport  Port=2
  VHAL_BatInTempErr_enum : Outport  Port=3
  VHAL_BatOutTemp_C : Outport  Port=4
  VHAL_COMPErr_enum : Outport  Port=5
  VHAL_EACProtectEnable_enum : Outport  Port=6
  VHAL_EWP3Err_enum : Outport  Port=7
  VHAL_EXV1Err_enum : Outport  Port=8
  VHAL_EXV2Err_enum : Outport  Port=9
  VHAL_FanErr_enum : Outport  Port=10
  VHAL_MotorInTemp_C : Outport  Port=11
  VHAL_MotorInTempErr_enum : Outport  Port=12
  VHAL_MotorOutTemp_C : Outport  Port=13
  VHAL_MotorOutTempErr_enum : Outport  Port=14
  VHAL_PTHighP_KPa : Outport  Port=15
  VHAL_PTHighPErr_enum : Outport  Port=16
  VHAL_PTHighTact_C : Outport  Port=17
  VHAL_PTHighTactErr_enum : Outport  Port=18
  VHAL_PTLowP1_KPa : Outport  Port=19
  VHAL_PTLowP1Err_enum : Outport  Port=20
  VHAL_PTLowP2_KPa : Outport  Port=21
  VHAL_PTLowP2Err_enum : Outport  Port=22
  VHAL_PTLowT1_C : Outport  Port=23
  VHAL_PTLowT1Err_enum : Outport  Port=24
  VHAL_PTLowT2_C : Outport  Port=25
  VHAL_PTLowT2Err_enum : Outport  Port=26
  VHAL_SOTXVErr_enum : Outport  Port=27
  VHAL_SOV1Err_enum : Outport  Port=28
  VHAL_SOV2Err_enum : Outport  Port=29
  VHAL_SOV3Err_enum : Outport  Port=30
  VHAL_Tamb_C : Outport  Port=31
  VHAL_TambErr_enum : Outport  Port=32
  wires:
  DT_CAN4_SG_Zone_Fr_THCM/1 -> [DT_CAN4_SG_Zone_Fr_THCM]
  [DT_CAN4_SG_Zone_Fr_THCM] -> bus_selector/1
  bus_selector/1 -> AGSErr/1(AGS_Err)  "<CAN4_AGS_Err>"
  AGSErr/1(VHAL_AGSErr_enum) -> VHAL_AGSErr_enum/1
  [DT_CAN4_SG_Zone_Fr_THCM] -> bus_selector1/1
  bus_selector1/1 -> BatInTemp/1(Bat_In_Temp)  "<CAN4_Bat_In_Temp>"
  BatInTemp/1(VHAL_BatInTemp_C) -> VHAL_BatInTemp_C/1
  [DT_CAN4_SG_Zone_Fr_THCM] -> bus_selector2/1
  bus_selector2/1 -> BatInTempErr/1(Bat_In_Temp_Err)  "<CAN4_Bat_In_Temp_Err>"
  BatInTempErr/1(VHAL_BatInTempErr_enum) -> VHAL_BatInTempErr_enum/1
  [DT_CAN4_SG_Zone_Fr_THCM] -> bus_selector3/1
  bus_selector3/1 -> BatOutTemp/1(Bat_Out_Temp)  "<CAN4_Bat_Out_Temp>"
  BatOutTemp/1(VHAL_BatOutTemp_C) -> VHAL_BatOutTemp_C/1
  [DT_CAN4_SG_Zone_Fr_THCM] -> bus_selector4/1
  bus_selector4/1 -> COMPErr/1(COMP_Err)  "<CAN4_COMP_Err>"
  COMPErr/1(VHAL_COMPErr_enum) -> VHAL_COMPErr_enum/1
  [DT_CAN4_SG_Zone_Fr_THCM] -> bus_selector5/1
  bus_selector5/1 -> EACProtectEnable/1(EACProtectEnable)  "<CAN4_EACProtectEnable>"
  EACProtectEnable/1(VHAL_EACProtectEnable_enum) -> VHAL_EACProtectEnable_enum/1
  [DT_CAN4_SG_Zone_Fr_THCM] -> bus_selector6/1
  bus_selector6/1 -> EWP3Err/1(EWP3_Err)  "<CAN4_EWP3_Err>"
  EWP3Err/1(VHAL_EWP3Err_enum) -> VHAL_EWP3Err_enum/1
  [DT_CAN4_SG_Zone_Fr_THCM] -> bus_selector7/1
  bus_selector7/1 -> EXV1Err/1(EXV1_Err)  "<CAN4_EXV1_Err>"
  EXV1Err/1(VHAL_EXV1Err_enum) -> VHAL_EXV1Err_enum/1
  [DT_CAN4_SG_Zone_Fr_THCM] -> bus_selector8/1
  bus_selector8/1 -> EXV2Err/1(EXV2_Err)  "<CAN4_EXV2_Err>"
  EXV2Err/1(VHAL_EXV2Err_enum) -> VHAL_EXV2Err_enum/1
  [DT_CAN4_SG_Zone_Fr_THCM] -> bus_selector9/1
  bus_selector9/1 -> FanErr/1(Fan_Err)  "<CAN4_Fan_Err>"
  FanErr/1(VHAL_FanErr_enum) -> VHAL_FanErr_enum/1
  [DT_CAN4_SG_Zone_Fr_THCM] -> bus_selector10/1
  bus_selector10/1 -> MotorInTemp/1(Motor_In_Temp)  "<CAN4_Motor_In_Temp>"
  MotorInTemp/1(VHAL_MotorInTemp_C) -> VHAL_MotorInTemp_C/1
  [DT_CAN4_SG_Zone_Fr_THCM] -> bus_selector11/1
  bus_selector11/1 -> MotorInTempErr/1(Motor_In_Temp_Err)  "<CAN4_Motor_In_Temp_Err>"
  MotorInTempErr/1(VHAL_MotorInTempErr_enum) -> VHAL_MotorInTempErr_enum/1
  [DT_CAN4_SG_Zone_Fr_THCM] -> bus_selector12/1
  bus_selector12/1 -> MotorOutTemp/1(Motor_Out_Temp)  "<CAN4_Motor_Out_Temp>"
  MotorOutTemp/1(VHAL_MotorOutTemp_C) -> VHAL_MotorOutTemp_C/1
  [DT_CAN4_SG_Zone_Fr_THCM] -> bus_selector13/1
  bus_selector13/1 -> MotorOutTempErr/1(Motor_Out_Temp_Err)  "<CAN4_Motor_Out_Temp_Err>"
  MotorOutTempErr/1(VHAL_MotorOutTempErr_enum) -> VHAL_MotorOutTempErr_enum/1
  [DT_CAN4_SG_Zone_Fr_THCM] -> bus_selector14/1
  bus_selector14/1 -> PTHighP/1(PT_High_P)  "<CAN4_PT_High_P>"
  PTHighP/1(VHAL_PTHighP_KPa) -> VHAL_PTHighP_KPa/1
  [DT_CAN4_SG_Zone_Fr_THCM] -> bus_selector15/1
  bus_selector15/1 -> PTHighPErr/1(PT_High_P_Err)  "<CAN4_PT_High_P_Err>"
  PTHighPErr/1(VHAL_PTHighPErr_enum) -> VHAL_PTHighPErr_enum/1
  [DT_CAN4_SG_Zone_Fr_THCM] -> bus_selector16/1
  bus_selector16/1 -> PTHighTact/1(PT_High_Tact)  "<CAN4_PT_High_Tact>"
  PTHighTact/1(VHAL_PTHighTact_C) -> VHAL_PTHighTact_C/1
  [DT_CAN4_SG_Zone_Fr_THCM] -> bus_selector17/1
  bus_selector17/1 -> PTHighTactErr/1(PT_High_Tact_Err)  "<CAN4_PT_High_Tact_Err>"
  PTHighTactErr/1(VHAL_PTHighTactErr_enum) -> VHAL_PTHighTactErr_enum/1
  [DT_CAN4_SG_Zone_Fr_THCM] -> bus_selector18/1
  bus_selector18/1 -> PTLowP1/1(PT_Low_P1)  "<CAN4_PT_Low_P1>"
  PTLowP1/1(VHAL_PTLowP1_KPa) -> VHAL_PTLowP1_KPa/1
  [DT_CAN4_SG_Zone_Fr_THCM] -> bus_selector19/1
  bus_selector19/1 -> PTLowP1Err/1(PT_Low_P1_Err)  "<CAN4_PT_Low_P1_Err>"
  PTLowP1Err/1(VHAL_PTLowP1Err_enum) -> VHAL_PTLowP1Err_enum/1
  [DT_CAN4_SG_Zone_Fr_THCM] -> bus_selector20/1
  bus_selector20/1 -> PTLowP2/1(PT_Low_P2)  "<CAN4_PT_Low_P2>"
  PTLowP2/1(VHAL_PTLowP2_KPa) -> VHAL_PTLowP2_KPa/1
  [DT_CAN4_SG_Zone_Fr_THCM] -> bus_selector21/1
  bus_selector21/1 -> PTLowP2Err/1(PT_Low_P2_Err)  "<CAN4_PT_Low_P2_Err>"
  PTLowP2Err/1(VHAL_PTLowP2Err_enum) -> VHAL_PTLowP2Err_enum/1
  [DT_CAN4_SG_Zone_Fr_THCM] -> bus_selector22/1
  bus_selector22/1 -> PTLowT1/1(PT_Low_T1)  "<CAN4_PT_Low_T1>"
  PTLowT1/1(VHAL_PTLowT1_C) -> VHAL_PTLowT1_C/1
  [DT_CAN4_SG_Zone_Fr_THCM] -> bus_selector23/1
  bus_selector23/1 -> PTLowT1Err/1(PT_Low_T1_Err)  "<CAN4_PT_Low_T1_Err>"
  PTLowT1Err/1(VHAL_PTLowT1Err_enum) -> VHAL_PTLowT1Err_enum/1
  [DT_CAN4_SG_Zone_Fr_THCM] -> bus_selector24/1
  bus_selector24/1 -> PTLowT2/1(PT_Low_T2)  "<CAN4_PT_Low_T2>"
  PTLowT2/1(VHAL_PTLowT2_C) -> VHAL_PTLowT2_C/1
  [DT_CAN4_SG_Zone_Fr_THCM] -> bus_selector25/1
  bus_selector25/1 -> PTLowT2Err/1(PT_Low_T2_Err)  "<CAN4_PT_Low_T2_Err>"
  PTLowT2Err/1(VHAL_PTLowT2Err_enum) -> VHAL_PTLowT2Err_enum/1
  [DT_CAN4_SG_Zone_Fr_THCM] -> bus_selector26/1
  bus_selector26/1 -> SOTXVErr/1(SOTXV_Err)  "<CAN4_SOTXV_Err>"
  SOTXVErr/1(VHAL_SOTXVErr_enum) -> VHAL_SOTXVErr_enum/1
  [DT_CAN4_SG_Zone_Fr_THCM] -> bus_selector27/1
  bus_selector27/1 -> SOV1Err/1(SOV1_Err)  "<CAN4_SOV1_Err>"
  SOV1Err/1(VHAL_SOV1Err_enum) -> VHAL_SOV1Err_enum/1
  [DT_CAN4_SG_Zone_Fr_THCM] -> bus_selector28/1
  bus_selector28/1 -> SOV2Err/1(SOV2_Err)  "<CAN4_SOV2_Err>"
  SOV2Err/1(VHAL_SOV2Err_enum) -> VHAL_SOV2Err_enum/1
  [DT_CAN4_SG_Zone_Fr_THCM] -> bus_selector29/1
  bus_selector29/1 -> SOV3Err/1(SOV3_Err)  "<CAN4_SOV3_Err>"
  SOV3Err/1(VHAL_SOV3Err_enum) -> VHAL_SOV3Err_enum/1
  [DT_CAN4_SG_Zone_Fr_THCM] -> bus_selector30/1
  bus_selector30/1 -> Tamb/1(Tamb)  "<CAN4_Tamb>"
  Tamb/1(VHAL_Tamb_C) -> VHAL_Tamb_C/1
  [DT_CAN4_SG_Zone_Fr_THCM] -> bus_selector31/1
  bus_selector31/1 -> TambErr/1(Tamb_Err)  "<CAN4_Tamb_Err>"
  TambErr/1(VHAL_TambErr_enum) -> VHAL_TambErr_enum/1

== system halin/HAL_IN/CAN5/TBOX1 ==
  DT_CAN5_SG_TBOX1 : Inport
  PowerOffTSet : Subsystem
  ReDoorLock : Subsystem
  ReOutsideMirror : Subsystem
  RePwrReqTbox : Subsystem
  RemoteACTemp : Subsystem
  RemoteAutoReq : Subsystem
  bus_selector : BusSelector  OutputSignals=CAN5_PowerOff_T_Set
  bus_selector1 : BusSelector  OutputSignals=CAN5_ReOutsideMirror
  bus_selector2 : BusSelector  OutputSignals=CAN5_Re_DoorLock
  bus_selector3 : BusSelector  OutputSignals=CAN5_Re_PwrReqTbox
  bus_selector4 : BusSelector  OutputSignals=CAN5_Remote_ACTemp
  bus_selector5 : BusSelector  OutputSignals=CAN5_Remote_AutoReq
  VHAL_PowerOffTSet_cnt : Outport
  VHAL_ReOutsideMirror_enum : Outport  Port=2
  VHAL_ReDoorLock_enum : Outport  Port=3
  VHAL_RePwrReqTbox_enum : Outport  Port=4
  VHAL_RemoteACTemp_C : Outport  Port=5
  VHAL_RemoteAutoReq_flg : Outport  Port=6
  wires:
  DT_CAN5_SG_TBOX1/1 -> [DT_CAN5_SG_TBOX1]
  [DT_CAN5_SG_TBOX1] -> bus_selector/1
  bus_selector/1 -> PowerOffTSet/1(PowerOff_T_Set)  "<CAN5_PowerOff_T_Set>"
  PowerOffTSet/1(VHAL_PowerOffTSet_cnt) -> VHAL_PowerOffTSet_cnt/1
  [DT_CAN5_SG_TBOX1] -> bus_selector1/1
  bus_selector1/1 -> ReOutsideMirror/1(ReOutsideMirror)  "<CAN5_ReOutsideMirror>"
  ReOutsideMirror/1(VHAL_ReOutsideMirror_enum) -> VHAL_ReOutsideMirror_enum/1
  [DT_CAN5_SG_TBOX1] -> bus_selector2/1
  bus_selector2/1 -> ReDoorLock/1(Re_DoorLock)  "<CAN5_Re_DoorLock>"
  ReDoorLock/1(VHAL_ReDoorLock_enum) -> VHAL_ReDoorLock_enum/1
  [DT_CAN5_SG_TBOX1] -> bus_selector3/1
  bus_selector3/1 -> RePwrReqTbox/1(Re_PwrReqTbox)  "<CAN5_Re_PwrReqTbox>"
  RePwrReqTbox/1(VHAL_RePwrReqTbox_enum) -> VHAL_RePwrReqTbox_enum/1
  [DT_CAN5_SG_TBOX1] -> bus_selector4/1
  bus_selector4/1 -> RemoteACTemp/1(Remote_ACTemp)  "<CAN5_Remote_ACTemp>"
  RemoteACTemp/1(VHAL_RemoteACTemp_C) -> VHAL_RemoteACTemp_C/1
  [DT_CAN5_SG_TBOX1] -> bus_selector5/1
  bus_selector5/1 -> RemoteAutoReq/1(Remote_AutoReq)  "<CAN5_Remote_AutoReq>"
  RemoteAutoReq/1(VHAL_RemoteAutoReq_flg) -> VHAL_RemoteAutoReq_flg/1

== system halin/HAL_IN/CAN5/VHAL_CANMsgInvalidTBOX1_flg ==
  Cast To Boolean13 : DataTypeConversion  OutDataTypeStr=boolean
  Constant : Constant  Value=TRUE
  Latch13 : hcu_lib/Basic_Blocks/Latch
  Switch13 : Switch  Criteria=u2 ~= 0
  Unit Delay : UnitDelay  SampleTime=-1  HasFrameUpgradeWarning=on
  UnitConverter : DataTypeConversion  OutDataTypeStr=boolean
  Out : Outport
  wires:
  Constant/1 -> Switch13/3
  Unit Delay/1 -> Cast To Boolean13/1
  Cast To Boolean13/1 -> Switch13/1, Latch13/1
  Switch13/1 -> UnitConverter/1
  Latch13/1 -> Switch13/2
  UnitConverter/1 -> Unit Delay/1, Out/1  "VHAL_CANMsgInvalidTBOX1_flg"

== system halin/HAL_IN/CAN1/ABM1/AirBagFailCmd ==
  AirBagFailCmd : Inport
  UnitConverter : DataTypeConversion  OutDataTypeStr=uint8
  VHAL_AirBagFailCmd_flg : Outport
  wires:
  UnitConverter/1 -> VHAL_AirBagFailCmd_flg/1
  AirBagFailCmd/1 -> UnitConverter/1

== system halin/HAL_IN/CAN1/ABM1/ChecksumABM1 ==
  Checksum_ABM1 : Inport
  UnitConverter : DataTypeConversion  OutDataTypeStr=uint8
  VHAL_ChecksumABM1_enum : Outport
  wires:
  UnitConverter/1 -> VHAL_ChecksumABM1_enum/1
  Checksum_ABM1/1 -> UnitConverter/1

== system halin/HAL_IN/CAN1/ABM1/CrashOutputSts ==
  CrashOutputSts : Inport
  UnitConverter : DataTypeConversion  OutDataTypeStr=uint8
  VHAL_CrashOutputSts_enum : Outport
  wires:
  UnitConverter/1 -> VHAL_CrashOutputSts_enum/1
  CrashOutputSts/1 -> UnitConverter/1

== system halin/HAL_IN/CAN1/ABM1/DriverSeatBeltCmd ==
  DriverSeatBeltCmd : Inport
  UnitConverter : DataTypeConversion  OutDataTypeStr=uint8
  VHAL_DriverSeatBeltCmd_flg : Outport
  wires:
  UnitConverter/1 -> VHAL_DriverSeatBeltCmd_flg/1
  DriverSeatBeltCmd/1 -> UnitConverter/1
